simulink library "xbsDSP48_r3"  (Simulink 5.0)
libraries: xbsIndex_r3 x429, xbsDSP48_r3 x2
(part 6 of 8)

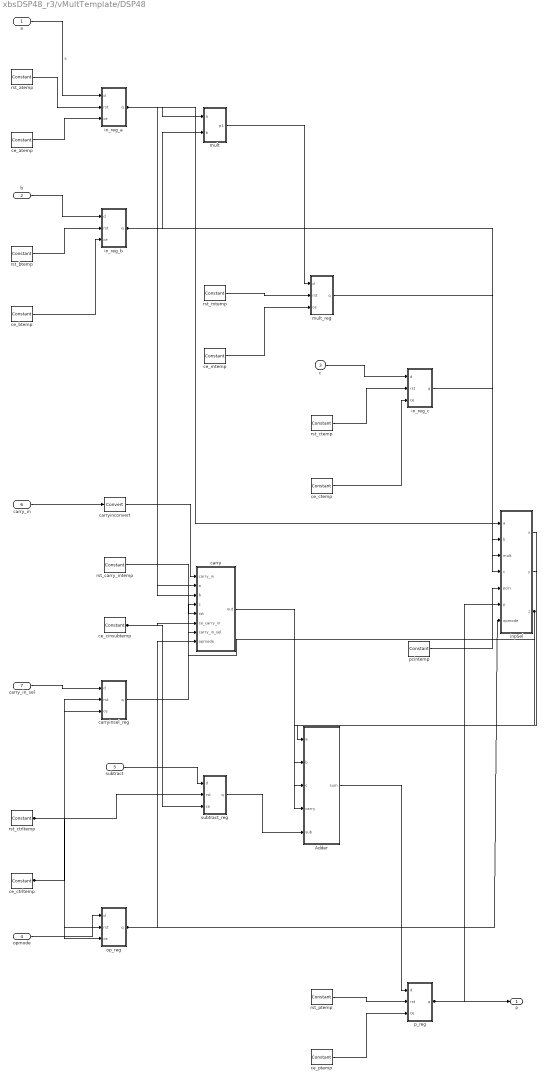
== system xbsDSP48_r3/vMultTemplate/DSP48 ==
  a : Inport
  b : Inport  Port=2
  c : Inport  Port=3
  opmode : Inport  Port=4
  subtract : Inport  Port=5
  carry_in : Inport  Port=6
  carry_in_sel : Inport  Port=7
  Adder : Subsystem
  carry : Subsystem
  carryinconvert : xbsIndex_r3/Convert  arith_type=Unsigned  n_bits=1  bin_pt=0  quantization=Truncate  overflow=Wrap  latency=0  explicit_period=off  period=1  dbl_ovrd=off  show_param=off  inserted_by_tool=off  pipeline=off
      settings: xl_area=[0, 0, 0, 0, 0, 0, 0]
  carryinsel_reg : Subsystem  mask{nreg=pipeline_carryinsel, pnreg=1}
      mask prompts: nreg "Number of registers"; pnreg "Previous number of register"
      mask init: same as xbsDSP48_r3/DSP48reg
      mask Display:
      | patch([0 iWidth iWidth 0],[0 0 iHeight iHeight] , bg);
      | patch(logoX,logoY , fg);
      | text(iCx-6,iCy,'z');
      | text(iCx,iCy+4,str);
      | port_label('input',1,'d');
      | port_label('input',2,'rst');
      | port_label('input',3,'ce');
      | port_label('output',1,'q');
      | plot([0 0 iWidth iWidth 0], [0 iHeight iHeight 0 0]);
  ce_atemp : xbsIndex_r3/Constant  const=1  equ=P=C  arith_type=Boolean  n_bits=1  bin_pt=0  opselect=C  inp2=PCIN>>17  opr=+  inp1=P  carry=CIN  iostate=0  explicit_period=on  period=2  dbl_ovrd=off
  ce_btemp : xbsIndex_r3/Constant  const=1  equ=P=C  arith_type=Boolean  n_bits=1  bin_pt=0  opselect=C  inp2=PCIN>>17  opr=+  inp1=P  carry=CIN  iostate=0  explicit_period=on  period=2  dbl_ovrd=off
  ce_cinsubtemp : xbsIndex_r3/Constant  const=1  equ=P=C  arith_type=Boolean  n_bits=1  bin_pt=0  opselect=C  inp2=PCIN>>17  opr=+  inp1=P  carry=CIN  iostate=0  explicit_period=on  period=2  dbl_ovrd=off
  ce_ctemp : xbsIndex_r3/Constant  const=1  equ=P=C  arith_type=Boolean  n_bits=1  bin_pt=0  opselect=C  inp2=PCIN>>17  opr=+  inp1=P  carry=CIN  iostate=0  explicit_period=on  period=2  dbl_ovrd=off
  ce_ctrltemp : xbsIndex_r3/Constant  const=1  arith_type=Boolean  n_bits=1  bin_pt=0  explicit_period=on  period=2  dbl_ovrd=off
  ce_mtemp : xbsIndex_r3/Constant  const=1  equ=P=C  arith_type=Boolean  n_bits=1  bin_pt=0  opselect=C  inp2=PCIN>>17  opr=+  inp1=P  carry=CIN  iostate=0  explicit_period=on  period=2  dbl_ovrd=off
  ce_ptemp : xbsIndex_r3/Constant  const=1  arith_type=Boolean  n_bits=1  bin_pt=0  explicit_period=on  period=2  dbl_ovrd=off
  in_reg_a : Subsystem  mask{nreg=pipeline_a-1, pnreg=1}
      mask prompts: nreg "Number of registers"; pnreg "Previous number of register"
      mask init: same as xbsDSP48_r3/DSP48reg
      mask Display:
      | patch([0 iWidth iWidth 0],[0 0 iHeight iHeight] , bg);
      | patch(logoX,logoY , fg);
      | text(iCx-6,iCy,'z');
      | text(iCx,iCy+4,str);
      | port_label('input',1,'d');
      | port_label('input',2,'rst');
      | port_label('input',3,'ce');
      | port_label('output',1,'q');
      | plot([0 0 iWidth iWidth 0], [0 iHeight iHeight 0 0]);
  in_reg_b : Subsystem  mask{nreg=pipeline_b- 1, pnreg=1}
      mask prompts: nreg "Number of registers"; pnreg "Previous number of register"
      mask init: same as xbsDSP48_r3/DSP48reg
      mask Display:
      | patch([0 iWidth iWidth 0],[0 0 iHeight iHeight] , bg);
      | patch(logoX,logoY , fg);
      | text(iCx-6,iCy,'z');
      | text(iCx,iCy+4,str);
      | port_label('input',1,'d');
      | port_label('input',2,'rst');
      | port_label('input',3,'ce');
      | port_label('output',1,'q');
      | plot([0 0 iWidth iWidth 0], [0 iHeight iHeight 0 0]);
  in_reg_c : Subsystem  mask{nreg=pipeline_c, pnreg=1}
      mask prompts: nreg "Number of registers"; pnreg "Previous number of register"
      mask init: same as xbsDSP48_r3/DSP48reg
      mask Display:
      | patch([0 iWidth iWidth 0],[0 0 iHeight iHeight] , bg);
      | patch(logoX,logoY , fg);
      | text(iCx-6,iCy,'z');
      | text(iCx,iCy+4,str);
      | port_label('input',1,'d');
      | port_label('input',2,'rst');
      | port_label('input',3,'ce');
      | port_label('output',1,'q');
      | plot([0 0 iWidth iWidth 0], [0 iHeight iHeight 0 0]);
  inpSel : Subsystem
  mult : Subsystem
  mult_reg : Subsystem  mask{nreg=pipeline_mult, pnreg=1}
      mask prompts: nreg "Number of registers"; pnreg "Previous number of register"
      mask init: same as xbsDSP48_r3/DSP48reg
      mask Display:
      | patch([0 iWidth iWidth 0],[0 0 iHeight iHeight] , bg);
      | patch(logoX,logoY , fg);
      | text(iCx-6,iCy,'z');
      | text(iCx,iCy+4,str);
      | port_label('input',1,'d');
      | port_label('input',2,'rst');
      | port_label('input',3,'ce');
      | port_label('output',1,'q');
      | plot([0 0 iWidth iWidth 0], [0 iHeight iHeight 0 0]);
  op_reg : Subsystem  mask{nreg=pipeline_opmode, pnreg=1}
      mask prompts: nreg "Number of registers"; pnreg "Previous number of register"
      mask init: same as xbsDSP48_r3/DSP48reg
      mask Display:
      | patch([0 iWidth iWidth 0],[0 0 iHeight iHeight] , bg);
      | patch(logoX,logoY , fg);
      | text(iCx-6,iCy,'z');
      | text(iCx,iCy+4,str);
      | port_label('input',1,'d');
      | port_label('input',2,'rst');
      | port_label('input',3,'ce');
      | port_label('output',1,'q');
      | plot([0 0 iWidth iWidth 0], [0 iHeight iHeight 0 0]);
  p_reg : Subsystem  mask{nreg=pipeline_p, pnreg=1}
      mask prompts: nreg "Number of registers"; pnreg "Previous number of register"
      mask init: same as xbsDSP48_r3/DSP48reg
      mask Display:
      | patch([0 iWidth iWidth 0],[0 0 iHeight iHeight] , bg);
      | patch(logoX,logoY , fg);
      | text(iCx-6,iCy,'z');
      | text(iCx,iCy+4,str);
      | port_label('input',1,'d');
      | port_label('input',2,'rst');
      | port_label('input',3,'ce');
      | port_label('output',1,'q');
      | plot([0 0 iWidth iWidth 0], [0 iHeight iHeight 0 0]);
  pcintemp : xbsIndex_r3/Constant  const=1  equ=P=C  arith_type="Signed  (2's comp)"  n_bits=48  bin_pt=0  opselect=C  inp2=PCIN>>17  opr=+  inp1=P  carry=CIN  iostate=0  explicit_period=on  period=2  dbl_ovrd=off
  rst_atemp : xbsIndex_r3/Constant  const=0  equ=P=C  arith_type=Boolean  n_bits=1  bin_pt=0  opselect=C  inp2=PCIN>>17  opr=+  inp1=P  carry=CIN  iostate=0  explicit_period=on  period=2  dbl_ovrd=off
  rst_btemp : xbsIndex_r3/Constant  const=0  equ=P=C  arith_type=Boolean  n_bits=1  bin_pt=0  opselect=C  inp2=PCIN>>17  opr=+  inp1=P  carry=CIN  iostate=0  explicit_period=on  period=2  dbl_ovrd=off
  rst_carry_intemp : xbsIndex_r3/Constant  const=0  equ=P=C  arith_type=Boolean  n_bits=1  bin_pt=0  opselect=C  inp2=PCIN>>17  opr=+  inp1=P  carry=CIN  iostate=0  explicit_period=on  period=2  dbl_ovrd=off
  rst_ctemp : xbsIndex_r3/Constant  const=0  equ=P=C  arith_type=Boolean  n_bits=1  bin_pt=0  opselect=C  inp2=PCIN>>17  opr=+  inp1=P  carry=CIN  iostate=0  explicit_period=on  period=2  dbl_ovrd=off
  rst_ctrltemp : xbsIndex_r3/Constant  const=0  arith_type=Boolean  n_bits=1  bin_pt=0  explicit_period=on  period=2  dbl_ovrd=off
  rst_mtemp : xbsIndex_r3/Constant  const=0  equ=P=C  arith_type=Boolean  n_bits=1  bin_pt=0  opselect=C  inp2=PCIN>>17  opr=+  inp1=P  carry=CIN  iostate=0  explicit_period=on  period=2  dbl_ovrd=off
  rst_ptemp : xbsIndex_r3/Constant  const=0  arith_type=Boolean  n_bits=1  bin_pt=0  explicit_period=on  period=2  dbl_ovrd=off
  subtract_reg : Subsystem  mask{nreg=pipeline_sub, pnreg=1}
      mask prompts: nreg "Number of registers"; pnreg "Previous number of register"
      mask init: same as xbsDSP48_r3/DSP48reg
      mask Display:
      | patch([0 iWidth iWidth 0],[0 0 iHeight iHeight] , bg);
      | patch(logoX,logoY , fg);
      | text(iCx-6,iCy,'z');
      | text(iCx,iCy+4,str);
      | port_label('input',1,'d');
      | port_label('input',2,'rst');
      | port_label('input',3,'ce');
      | port_label('output',1,'q');
      | plot([0 0 iWidth iWidth 0], [0 iHeight iHeight 0 0]);
  P : Outport
  wires:
  ce_cinsubtemp/1 -> subtract_reg/3(ce), carry/6(ce_carry_in)
  ce_ctrltemp/1 -> op_reg/3(ce), carryinsel_reg/3(ce)
  rst_ctrltemp/1 -> carryinsel_reg/2(rst), subtract_reg/2(rst), op_reg/2(rst)
  p_reg/1(q) -> inpSel/6(p), P/1
  in_reg_b/1(q) -> carry/3(b), inpSel/2(b), mult/2(b)
  op_reg/1(q) -> carry/8(opmode), inpSel/7(opmode)
  inpSel/3(z) -> carry/4(z), Adder/3(c)
  in_reg_a/1(q) -> inpSel/1(a), carry/2(a), mult/1(a)
  pcintemp/1 -> inpSel/5(pcin)
  ce_mtemp/1 -> mult_reg/3(ce)
  ce_ptemp/1 -> p_reg/3(ce)
  ce_ctemp/1 -> in_reg_c/3(ce)
  ce_btemp/1 -> in_reg_b/3(ce)
  ce_atemp/1 -> in_reg_a/3(ce)
  rst_carry_intemp/1 -> carry/5(rst)
  rst_mtemp/1 -> mult_reg/2(rst)
  rst_ptemp/1 -> p_reg/2(rst)
  rst_ctemp/1 -> in_reg_c/2(rst)
  rst_btemp/1 -> in_reg_b/2(rst)
  rst_atemp/1 -> in_reg_a/2(rst)
  b/1 -> in_reg_b/1(d)
  carryinsel_reg/1(q) -> carry/7(carry_in_sel)
  carry_in_sel/1 -> carryinsel_reg/1(d)
  carry_in/1 -> carryinconvert/1
  opmode/1 -> op_reg/1(d)
  a/1 -> in_reg_a/1(d)  "a"
  subtract/1 -> subtract_reg/1(d)
  carry/1(out) -> Adder/4(carry)
  subtract_reg/1(q) -> Adder/5(sub)
  Adder/1(sum) -> p_reg/1(d)
  inpSel/2(y) -> Adder/2(b)
  inpSel/1(x) -> Adder/1(a)
  mult_reg/1(q) -> inpSel/3(mult)
  mult/1(p1) -> mult_reg/1(d)
  in_reg_c/1(q) -> inpSel/4(c)
  carryinconvert/1 -> carry/1(carry_in)
  c/1 -> in_reg_c/1(d)
